simulink model "momentum_dump_test_rev2_simple"  (R2016b)
settings: Solver=VariableStepAuto  StartTime=0.0  StopTime=100  MinStep=0.001  RelTol=1e-3
values from neighbouring files (symbols this model uses):
  fsw_params = init_fsw_params()    [momentum_unload_test_init.m]
settings Model: Creator=evich  LastModifiedBy=evich

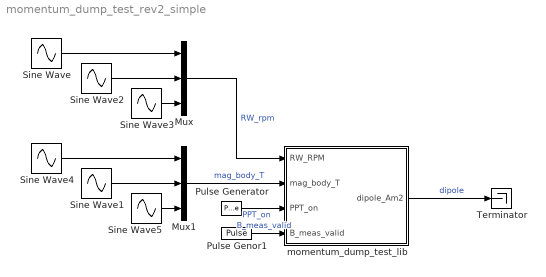
== system momentum_dump_test_rev2_simple ==
  Mux : Mux  Inputs=3
  Mux1 : Mux  Inputs=3
  Pulse Generator : DiscretePulseGenerator  PulseType=Time based  Period=fsw_params.actuators.ppt.sync_pulse  PulseWidth=fsw_params.actuators.ppt.t_charge_pct
  Pulse Genor1 : DiscretePulseGenerator  PulseType=Time based  Period=10  PulseWidth=sim_params.sensors.magnetometer.valid_pct
  Sine Wave : Sin  Amplitude=5  Frequency=3  SampleTime=0
  Sine Wave1 : Sin  Amplitude=0.0001  SampleTime=0
  Sine Wave2 : Sin  Amplitude=20  Frequency=0.5  SampleTime=0
  Sine Wave3 : Sin  Amplitude=4  SampleTime=0
  Sine Wave4 : Sin  Amplitude=0.0003  Frequency=1.5  SampleTime=0
  Sine Wave5 : Sin  Amplitude=0.00009  Frequency=2  SampleTime=0
  Terminator : Terminator
  momentum_dump_test_lib : Subsystem
  wires:
  Pulse Generator/1 -> momentum_dump_test_lib/3(PPT_on)  "PPT_on"
  Pulse Genor1/1 -> momentum_dump_test_lib/4(B_meas_valid)  "B_meas_valid"
  momentum_dump_test_lib/1(dipole_Am2) -> Terminator/1  "dipole"
  Sine Wave/1 -> Mux/1
  Sine Wave2/1 -> Mux/2
  Sine Wave3/1 -> Mux/3
  Mux/1 -> momentum_dump_test_lib/1(RW_RPM)  "RW_rpm"
  Mux1/1 -> momentum_dump_test_lib/2(mag_body_T)  "mag_body_T"
  Sine Wave1/1 -> Mux1/2
  Sine Wave4/1 -> Mux1/1
  Sine Wave5/1 -> Mux1/3

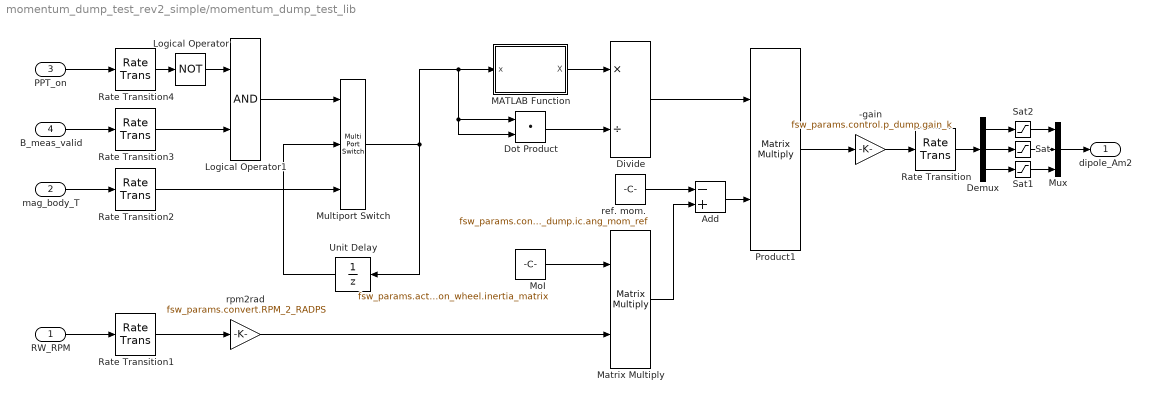
== system momentum_dump_test_rev2_simple/momentum_dump_test_lib ==
  RW_RPM : Inport
  mag_body_T : Inport  Port=2
  PPT_on : Inport  Port=3
  B_meas_valid : Inport  Port=4
  -gain : Gain  Gain=fsw_params.control.p_dump.gain_k
  Add : Sum  Inputs=-+
  Demux : Demux  Outputs=3
  Divide : Product  Inputs=*/
  Dot Product : DotProduct  InputSameDT=on  OutDataTypeStr=Inherit: Inherit via internal rule
  Logical Operator : Logic  Operator=NOT  AllPortsSameDT=off  OutDataTypeStr=boolean
  Logical Operator1 : Logic  AllPortsSameDT=off  OutDataTypeStr=boolean
  MATLAB Function : MATLAB Function  TreatAsAtomicUnit=on
  Matrix Multiply : Product  Inputs=**  Multiplication=Matrix(*)
  MoI : Constant  Value=fsw_params.actuators.reaction_wheel.inertia_matrix
  Multiport Switch : MultiPortSwitch  DataPortOrder=Zero-based contiguous  Inputs=2
  Mux : Mux  Inputs=3
  Product1 : Product  Inputs=**  Multiplication=Matrix(*)
  Rate Transition : RateTransition  X0=fsw_params.control.p_dump.ic.rt_dipole_Am2
  Rate Transition1 : RateTransition  X0=fsw_params.control.p_dump.ic.rt_w_body_radps  OutPortSampleTime=fsw_params.control.p_dump.sample_time_s
  Rate Transition2 : RateTransition  X0=fsw_params.control.p_dump.ic.rt_mag_body_T  OutPortSampleTime=fsw_params.control.p_dump.sample_time_s
  Rate Transition3 : RateTransition  X0=fsw_params.control.p_dump.ic.rt_B_meas_valid  OutPortSampleTime=fsw_params.control.p_dump.sample_time_s
  Rate Transition4 : RateTransition  X0=fsw_params.control.p_dump.ic.rt_PPT_on  OutPortSampleTime=fsw_params.control.p_dump.sample_time_s
  Sat : Saturate  UpperLimit=fsw_params.actuators.magnetorquer.max_dipole_y  LowerLimit=-fsw_params.actuators.magnetorquer.max_dipole_y
  Sat1 : Saturate  UpperLimit=fsw_params.actuators.magnetorquer.max_dipole_z  LowerLimit=-fsw_params.actuators.magnetorquer.max_dipole_z
  Sat2 : Saturate  UpperLimit=fsw_params.actuators.magnetorquer.max_dipole_x  LowerLimit=-fsw_params.actuators.magnetorquer.max_dipole_x
  Unit Delay : UnitDelay  InitialCondition=fsw_params.control.p_dump.ic.delay  SampleTime=-1
  ref. mom. : Constant  Value=fsw_params.control.p_dump.ic.ang_mom_ref
  rpm2rad : Gain  Gain=fsw_params.convert.RPM_2_RADPS
  dipole_Am2 : Outport
  wires:
  Dot Product/1 -> Divide/2
  ref. mom./1 -> Add/1
  Matrix Multiply/1 -> Add/2
  MATLAB Function/1(X) -> Divide/1
  MoI/1 -> Matrix Multiply/1
  Multiport Switch/1 -> MATLAB Function/1(x), Dot Product/2, Dot Product/1, Unit Delay/1
  rpm2rad/1 -> Matrix Multiply/2
  Add/1 -> Product1/2
  Divide/1 -> Product1/1
  Product1/1 -> -gain/1
  Logical Operator1/1 -> Multiport Switch/1
  Logical Operator/1 -> Logical Operator1/1
  Rate Transition3/1 -> Logical Operator1/2
  Rate Transition4/1 -> Logical Operator/1
  Rate Transition2/1 -> Multiport Switch/3
  Unit Delay/1 -> Multiport Switch/2
  PPT_on/1 -> Rate Transition4/1
  B_meas_valid/1 -> Rate Transition3/1
  mag_body_T/1 -> Rate Transition2/1
  RW_RPM/1 -> Rate Transition1/1
  Rate Transition1/1 -> rpm2rad/1
  Rate Transition/1 -> Demux/1
  Demux/2 -> Sat/1
  Demux/1 -> Sat2/1
  Demux/3 -> Sat1/1
  Sat1/1 -> Mux/3
  Sat/1 -> Mux/2
  Sat2/1 -> Mux/1
  Mux/1 -> dipole_Am2/1
  -gain/1 -> Rate Transition/1

== matlab function momentum_dump_test_rev2_simple/momentum_dump_test_lib/MATLAB Function ==
  data: x input; X output
function X   = skew( x )
% UW HuskySat-1, ADCS Subsystem
% Last Update: E. Hansen 12.8.2017

%Transforms a vector into a skew symmetric matrix (Levi-Civita)
%--------------------------------------------------------------------------

X = [0 -x(3) x(2);x(3) 0 -x(1);-x(2) x(1) 0];
